simulink model "imu"  (R2023a)
settings: Solver=ode4  StartTime=0.0  StopTime=10.0  FixedStep=dt  RelTol=1e-3
undefined symbols (not defined in the file or in its folder): dt
libraries: simulink x1
settings Model: Creator=ndelurgio  LastModifiedBy=ndelurgio

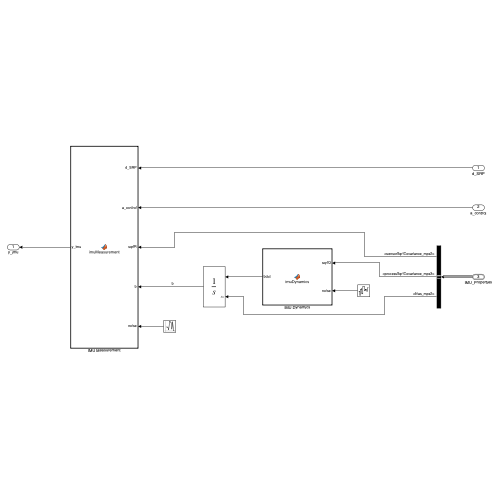
[thumbnail: Simulink's stored preview of the top-level diagram]
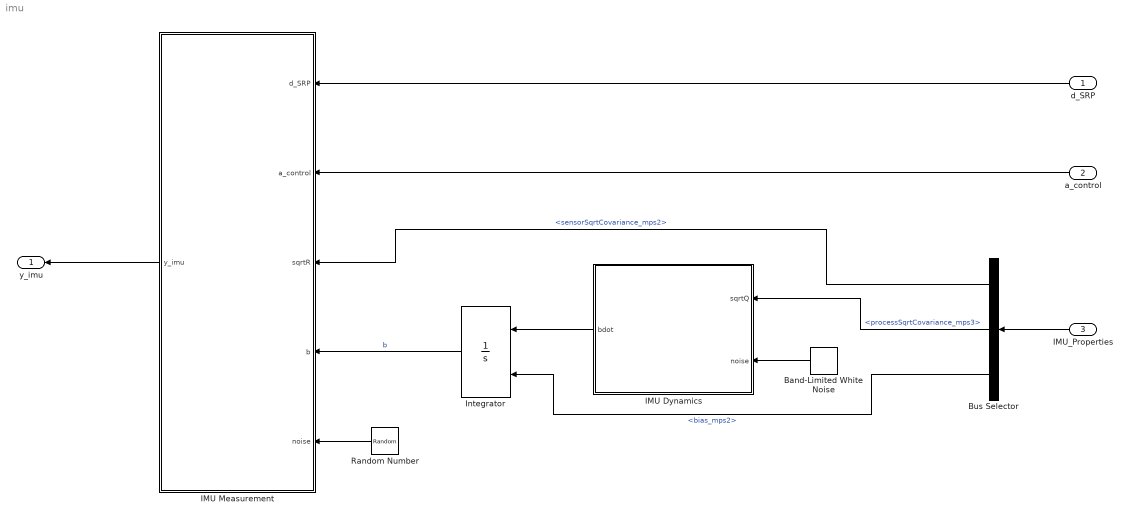
== system imu ==
  d_SRP : Inport  PortDimensions=3
  a_control : Inport  Port=2  PortDimensions=3
  IMU_Properties : Inport  Port=3  OutDataTypeStr=Bus: imu
  Band-Limited White Noise : simulink/Sources/Band-Limited White Noise  Cov=[1;1;1]  Ts=dt  seed=[21;56;23341]
  Bus Selector : BusSelector  OutputSignals=sensorSqrtCovariance_mps2,processSqrtCovariance_mps3,bias_mps2
  IMU Dynamics : MATLAB Function  TreatAsAtomicUnit=on
  IMU Measurement : MATLAB Function  TreatAsAtomicUnit=on
  Integrator : Integrator  InitialConditionSource=external
  Random Number : RandomNumber  Mean=[0;0;0]  Variance=[1;1;1]  Seed=[50;60;70]  SampleTime=dt
  y_imu : Outport
  wires:
  IMU_Properties/1 -> Bus Selector/1
  Bus Selector/2 -> IMU Dynamics/1(sqrtQ)  "<processSqrtCovariance_mps3>"
  Bus Selector/3 -> Integrator/2  "<bias_mps2>"
  IMU Dynamics/1(bdot) -> Integrator/1
  Integrator/1 -> IMU Measurement/4(b)  "b"
  Bus Selector/1 -> IMU Measurement/3(sqrtR)  "<sensorSqrtCovariance_mps2>"
  a_control/1 -> IMU Measurement/2(a_control)
  d_SRP/1 -> IMU Measurement/1(d_SRP)
  IMU Measurement/1(y_imu) -> y_imu/1
  Random Number/1 -> IMU Measurement/5(noise)
  Band-Limited White Noise/1 -> IMU Dynamics/2(noise)

== matlab function imu/IMU Measurement ==
  data: d_SRP input; y_imu output; a_control input; sqrtR input; b input; noise input
function y_imu = imuMeasurement(d_SRP,a_control,sqrtR,b,noise)

y_imu = imuMeasurement(d_SRP,a_control,b,sqrtR,noise);

end

== matlab function imu/IMU Dynamics ==
  data: sqrtQ input; bdot output; noise input
function bdot = imuDynamics(sqrtQ,noise)

bdot = imuDynamics(sqrtQ,noise);

end
